simulink model "natural_circulation_simscape_correct"  (R2018b)
settings: Solver=VariableStepAuto  StartTime=0.0  StopTime=100000  RelTol=1e-3  AbsTol=1e-3  EnableMultiTasking=on
values from neighbouring files (symbols this model uses):
  air_height_air = 5    [hub_initialize.m]
  cp = 1.22    [hub_initialize.m]
  density_air = 293./(temp_air)    [hub_initialize.m]
  density_nak = [0.866 0.855 0.749]    [hub_initialize.m]
  height_final = height_list(i)    [parametric_simulation.m]
  temp = density_nak_temperature'    [hub_initialize.m]
  temp_air = 293:10:700    [hub_initialize.m]
libraries: fl_lib x43, nesl_utility x9, SimscapeFluids_lib x3
(part 2 of 2)

== system natural_circulation_simscape_correct/Subsystem ==
